simulink model "UART"  (R2025a)
settings: Solver=FixedStepAuto  StartTime=0.0  StopTime=10  FixedStep=1e-6  RelTol=1e-3
undefined symbols (not defined in the file): Bit_1, Bit_2, Bit_3, Bit_4, Bit_5, Bit_6, Bit_7, Bit_8
libraries: simulink_extras x158, fl_lib x17, nesl_utility x8, simulink x7
(part 6 of 6)

== system UART/Subsystem1/Baudrate Generator/BPS/Subsystem1 ==
  Data : Inport
  Store : Inport  Port=2
  Clock : Inport  Port=3
  Clear : Inport  Port=4
  AND : Logic  IconShape=distinctive  AllPortsSameDT=off  OutDataTypeStr=boolean
  AND1 : Logic  IconShape=distinctive  AllPortsSameDT=off  OutDataTypeStr=boolean
  D Flip-Flop : simulink_extras/Flip Flops/D Flip-Flop
  NOT : Logic  Operator=NOT  IconShape=distinctive  AllPortsSameDT=off  OutDataTypeStr=boolean
  NOT1 : Logic  Operator=NOT  IconShape=distinctive  AllPortsSameDT=off  OutDataTypeStr=boolean
  OR : Logic  Operator=OR  IconShape=distinctive  AllPortsSameDT=off  OutDataTypeStr=boolean
  Q : Outport
  !Q : Outport  Port=2
  wires:
  AND1/1 -> OR/2
  AND/1 -> OR/1
  D Flip-Flop/1 -> Q/1, AND1/2
  NOT/1 -> AND1/1
  Store/1 -> AND/2, NOT/1
  Clock/1 -> D Flip-Flop/2
  Data/1 -> AND/1
  OR/1 -> D Flip-Flop/1
  D Flip-Flop/2 -> !Q/1
  Clear/1 -> NOT1/1
  NOT1/1 -> D Flip-Flop/3

== system UART/Subsystem1/Baudrate Generator/BPS/Subsystem2 ==
  Data : Inport
  Store : Inport  Port=2
  Clock : Inport  Port=3
  Clear : Inport  Port=4
  AND : Logic  IconShape=distinctive  AllPortsSameDT=off  OutDataTypeStr=boolean
  AND1 : Logic  IconShape=distinctive  AllPortsSameDT=off  OutDataTypeStr=boolean
  D Flip-Flop : simulink_extras/Flip Flops/D Flip-Flop
  NOT : Logic  Operator=NOT  IconShape=distinctive  AllPortsSameDT=off  OutDataTypeStr=boolean
  NOT1 : Logic  Operator=NOT  IconShape=distinctive  AllPortsSameDT=off  OutDataTypeStr=boolean
  OR : Logic  Operator=OR  IconShape=distinctive  AllPortsSameDT=off  OutDataTypeStr=boolean
  Q : Outport
  !Q : Outport  Port=2
  wires:
  AND1/1 -> OR/2
  AND/1 -> OR/1
  D Flip-Flop/1 -> Q/1, AND1/2
  NOT/1 -> AND1/1
  Store/1 -> AND/2, NOT/1
  Clock/1 -> D Flip-Flop/2
  Data/1 -> AND/1
  OR/1 -> D Flip-Flop/1
  D Flip-Flop/2 -> !Q/1
  Clear/1 -> NOT1/1
  NOT1/1 -> D Flip-Flop/3

== system UART/Subsystem1/Baudrate Generator/BPS/Subsystem3 ==
  Data : Inport
  Store : Inport  Port=2
  Clock : Inport  Port=3
  Clear : Inport  Port=4
  AND : Logic  IconShape=distinctive  AllPortsSameDT=off  OutDataTypeStr=boolean
  AND1 : Logic  IconShape=distinctive  AllPortsSameDT=off  OutDataTypeStr=boolean
  D Flip-Flop : simulink_extras/Flip Flops/D Flip-Flop
  NOT : Logic  Operator=NOT  IconShape=distinctive  AllPortsSameDT=off  OutDataTypeStr=boolean
  NOT1 : Logic  Operator=NOT  IconShape=distinctive  AllPortsSameDT=off  OutDataTypeStr=boolean
  OR : Logic  Operator=OR  IconShape=distinctive  AllPortsSameDT=off  OutDataTypeStr=boolean
  Q : Outport
  !Q : Outport  Port=2
  wires:
  AND1/1 -> OR/2
  AND/1 -> OR/1
  D Flip-Flop/1 -> Q/1, AND1/2
  NOT/1 -> AND1/1
  Store/1 -> AND/2, NOT/1
  Clock/1 -> D Flip-Flop/2
  Data/1 -> AND/1
  OR/1 -> D Flip-Flop/1
  D Flip-Flop/2 -> !Q/1
  Clear/1 -> NOT1/1
  NOT1/1 -> D Flip-Flop/3

== system UART/Subsystem1/Baudrate Generator/BPS/Subsystem4 ==
  Data : Inport
  Store : Inport  Port=2
  Clock : Inport  Port=3
  Clear : Inport  Port=4
  AND : Logic  IconShape=distinctive  AllPortsSameDT=off  OutDataTypeStr=boolean
  AND1 : Logic  IconShape=distinctive  AllPortsSameDT=off  OutDataTypeStr=boolean
  D Flip-Flop : simulink_extras/Flip Flops/D Flip-Flop
  NOT : Logic  Operator=NOT  IconShape=distinctive  AllPortsSameDT=off  OutDataTypeStr=boolean
  NOT1 : Logic  Operator=NOT  IconShape=distinctive  AllPortsSameDT=off  OutDataTypeStr=boolean
  OR : Logic  Operator=OR  IconShape=distinctive  AllPortsSameDT=off  OutDataTypeStr=boolean
  Q : Outport
  !Q : Outport  Port=2
  wires:
  AND1/1 -> OR/2
  AND/1 -> OR/1
  D Flip-Flop/1 -> Q/1, AND1/2
  NOT/1 -> AND1/1
  Store/1 -> AND/2, NOT/1
  Clock/1 -> D Flip-Flop/2
  Data/1 -> AND/1
  OR/1 -> D Flip-Flop/1
  D Flip-Flop/2 -> !Q/1
  Clear/1 -> NOT1/1
  NOT1/1 -> D Flip-Flop/3

== system UART/Subsystem1/Baudrate Generator/BPS/Subsystem5 ==
  Data : Inport
  Store : Inport  Port=2
  Clock : Inport  Port=3
  Clear : Inport  Port=4
  AND : Logic  IconShape=distinctive  AllPortsSameDT=off  OutDataTypeStr=boolean
  AND1 : Logic  IconShape=distinctive  AllPortsSameDT=off  OutDataTypeStr=boolean
  D Flip-Flop : simulink_extras/Flip Flops/D Flip-Flop
  NOT : Logic  Operator=NOT  IconShape=distinctive  AllPortsSameDT=off  OutDataTypeStr=boolean
  NOT1 : Logic  Operator=NOT  IconShape=distinctive  AllPortsSameDT=off  OutDataTypeStr=boolean
  OR : Logic  Operator=OR  IconShape=distinctive  AllPortsSameDT=off  OutDataTypeStr=boolean
  Q : Outport
  !Q : Outport  Port=2
  wires:
  AND1/1 -> OR/2
  AND/1 -> OR/1
  D Flip-Flop/1 -> Q/1, AND1/2
  NOT/1 -> AND1/1
  Store/1 -> AND/2, NOT/1
  Clock/1 -> D Flip-Flop/2
  Data/1 -> AND/1
  OR/1 -> D Flip-Flop/1
  D Flip-Flop/2 -> !Q/1
  Clear/1 -> NOT1/1
  NOT1/1 -> D Flip-Flop/3

== system UART/Subsystem1/Baudrate Generator/BPS/Subsystem6 ==
  Data : Inport
  Store : Inport  Port=2
  Clock : Inport  Port=3
  Clear : Inport  Port=4
  AND : Logic  IconShape=distinctive  AllPortsSameDT=off  OutDataTypeStr=boolean
  AND1 : Logic  IconShape=distinctive  AllPortsSameDT=off  OutDataTypeStr=boolean
  D Flip-Flop : simulink_extras/Flip Flops/D Flip-Flop
  NOT : Logic  Operator=NOT  IconShape=distinctive  AllPortsSameDT=off  OutDataTypeStr=boolean
  NOT1 : Logic  Operator=NOT  IconShape=distinctive  AllPortsSameDT=off  OutDataTypeStr=boolean
  OR : Logic  Operator=OR  IconShape=distinctive  AllPortsSameDT=off  OutDataTypeStr=boolean
  Q : Outport
  !Q : Outport  Port=2
  wires:
  AND1/1 -> OR/2
  AND/1 -> OR/1
  D Flip-Flop/1 -> Q/1, AND1/2
  NOT/1 -> AND1/1
  Store/1 -> AND/2, NOT/1
  Clock/1 -> D Flip-Flop/2
  Data/1 -> AND/1
  OR/1 -> D Flip-Flop/1
  D Flip-Flop/2 -> !Q/1
  Clear/1 -> NOT1/1
  NOT1/1 -> D Flip-Flop/3

== system UART/Subsystem1/Baudrate Generator/BPS/Subsystem7 ==
  Data : Inport
  Store : Inport  Port=2
  Clock : Inport  Port=3
  Clear : Inport  Port=4
  AND : Logic  IconShape=distinctive  AllPortsSameDT=off  OutDataTypeStr=boolean
  AND1 : Logic  IconShape=distinctive  AllPortsSameDT=off  OutDataTypeStr=boolean
  D Flip-Flop : simulink_extras/Flip Flops/D Flip-Flop
  NOT : Logic  Operator=NOT  IconShape=distinctive  AllPortsSameDT=off  OutDataTypeStr=boolean
  NOT1 : Logic  Operator=NOT  IconShape=distinctive  AllPortsSameDT=off  OutDataTypeStr=boolean
  OR : Logic  Operator=OR  IconShape=distinctive  AllPortsSameDT=off  OutDataTypeStr=boolean
  Q : Outport
  !Q : Outport  Port=2
  wires:
  AND1/1 -> OR/2
  AND/1 -> OR/1
  D Flip-Flop/1 -> Q/1, AND1/2
  NOT/1 -> AND1/1
  Store/1 -> AND/2, NOT/1
  Clock/1 -> D Flip-Flop/2
  Data/1 -> AND/1
  OR/1 -> D Flip-Flop/1
  D Flip-Flop/2 -> !Q/1
  Clear/1 -> NOT1/1
  NOT1/1 -> D Flip-Flop/3

== system UART/Subsystem1/Baudrate Generator/BPS/Subsystem8 ==
  Data : Inport
  Store : Inport  Port=2
  Clock : Inport  Port=3
  Clear : Inport  Port=4
  AND : Logic  IconShape=distinctive  AllPortsSameDT=off  OutDataTypeStr=boolean
  AND1 : Logic  IconShape=distinctive  AllPortsSameDT=off  OutDataTypeStr=boolean
  D Flip-Flop : simulink_extras/Flip Flops/D Flip-Flop
  NOT : Logic  Operator=NOT  IconShape=distinctive  AllPortsSameDT=off  OutDataTypeStr=boolean
  NOT1 : Logic  Operator=NOT  IconShape=distinctive  AllPortsSameDT=off  OutDataTypeStr=boolean
  OR : Logic  Operator=OR  IconShape=distinctive  AllPortsSameDT=off  OutDataTypeStr=boolean
  Q : Outport
  !Q : Outport  Port=2
  wires:
  AND1/1 -> OR/2
  AND/1 -> OR/1
  D Flip-Flop/1 -> Q/1, AND1/2
  NOT/1 -> AND1/1
  Store/1 -> AND/2, NOT/1
  Clock/1 -> D Flip-Flop/2
  Data/1 -> AND/1
  OR/1 -> D Flip-Flop/1
  D Flip-Flop/2 -> !Q/1
  Clear/1 -> NOT1/1
  NOT1/1 -> D Flip-Flop/3

== system UART/Subsystem1/Baudrate Generator/BR/Subsystem1 ==
  Data : Inport
  Store : Inport  Port=2
  Clock : Inport  Port=3
  Clear : Inport  Port=4
  AND : Logic  IconShape=distinctive  AllPortsSameDT=off  OutDataTypeStr=boolean
  AND1 : Logic  IconShape=distinctive  AllPortsSameDT=off  OutDataTypeStr=boolean
  D Flip-Flop : simulink_extras/Flip Flops/D Flip-Flop
  NOT : Logic  Operator=NOT  IconShape=distinctive  AllPortsSameDT=off  OutDataTypeStr=boolean
  NOT1 : Logic  Operator=NOT  IconShape=distinctive  AllPortsSameDT=off  OutDataTypeStr=boolean
  OR : Logic  Operator=OR  IconShape=distinctive  AllPortsSameDT=off  OutDataTypeStr=boolean
  Q : Outport
  !Q : Outport  Port=2
  wires:
  AND1/1 -> OR/2
  AND/1 -> OR/1
  D Flip-Flop/1 -> Q/1, AND1/2
  NOT/1 -> AND1/1
  Store/1 -> AND/2, NOT/1
  Clock/1 -> D Flip-Flop/2
  Data/1 -> AND/1
  OR/1 -> D Flip-Flop/1
  D Flip-Flop/2 -> !Q/1
  Clear/1 -> NOT1/1
  NOT1/1 -> D Flip-Flop/3

== system UART/Subsystem1/Baudrate Generator/BR/Subsystem2 ==
  Data : Inport
  Store : Inport  Port=2
  Clock : Inport  Port=3
  Clear : Inport  Port=4
  AND : Logic  IconShape=distinctive  AllPortsSameDT=off  OutDataTypeStr=boolean
  AND1 : Logic  IconShape=distinctive  AllPortsSameDT=off  OutDataTypeStr=boolean
  D Flip-Flop : simulink_extras/Flip Flops/D Flip-Flop
  NOT : Logic  Operator=NOT  IconShape=distinctive  AllPortsSameDT=off  OutDataTypeStr=boolean
  NOT1 : Logic  Operator=NOT  IconShape=distinctive  AllPortsSameDT=off  OutDataTypeStr=boolean
  OR : Logic  Operator=OR  IconShape=distinctive  AllPortsSameDT=off  OutDataTypeStr=boolean
  Q : Outport
  !Q : Outport  Port=2
  wires:
  AND1/1 -> OR/2
  AND/1 -> OR/1
  D Flip-Flop/1 -> Q/1, AND1/2
  NOT/1 -> AND1/1
  Store/1 -> AND/2, NOT/1
  Clock/1 -> D Flip-Flop/2
  Data/1 -> AND/1
  OR/1 -> D Flip-Flop/1
  D Flip-Flop/2 -> !Q/1
  Clear/1 -> NOT1/1
  NOT1/1 -> D Flip-Flop/3

== system UART/Subsystem1/Baudrate Generator/BR/Subsystem3 ==
  Data : Inport
  Store : Inport  Port=2
  Clock : Inport  Port=3
  Clear : Inport  Port=4
  AND : Logic  IconShape=distinctive  AllPortsSameDT=off  OutDataTypeStr=boolean
  AND1 : Logic  IconShape=distinctive  AllPortsSameDT=off  OutDataTypeStr=boolean
  D Flip-Flop : simulink_extras/Flip Flops/D Flip-Flop
  NOT : Logic  Operator=NOT  IconShape=distinctive  AllPortsSameDT=off  OutDataTypeStr=boolean
  NOT1 : Logic  Operator=NOT  IconShape=distinctive  AllPortsSameDT=off  OutDataTypeStr=boolean
  OR : Logic  Operator=OR  IconShape=distinctive  AllPortsSameDT=off  OutDataTypeStr=boolean
  Q : Outport
  !Q : Outport  Port=2
  wires:
  AND1/1 -> OR/2
  AND/1 -> OR/1
  D Flip-Flop/1 -> Q/1, AND1/2
  NOT/1 -> AND1/1
  Store/1 -> AND/2, NOT/1
  Clock/1 -> D Flip-Flop/2
  Data/1 -> AND/1
  OR/1 -> D Flip-Flop/1
  D Flip-Flop/2 -> !Q/1
  Clear/1 -> NOT1/1
  NOT1/1 -> D Flip-Flop/3

== system UART/Subsystem1/Baudrate Generator/BR/Subsystem4 ==
  Data : Inport
  Store : Inport  Port=2
  Clock : Inport  Port=3
  Clear : Inport  Port=4
  AND : Logic  IconShape=distinctive  AllPortsSameDT=off  OutDataTypeStr=boolean
  AND1 : Logic  IconShape=distinctive  AllPortsSameDT=off  OutDataTypeStr=boolean
  D Flip-Flop : simulink_extras/Flip Flops/D Flip-Flop
  NOT : Logic  Operator=NOT  IconShape=distinctive  AllPortsSameDT=off  OutDataTypeStr=boolean
  NOT1 : Logic  Operator=NOT  IconShape=distinctive  AllPortsSameDT=off  OutDataTypeStr=boolean
  OR : Logic  Operator=OR  IconShape=distinctive  AllPortsSameDT=off  OutDataTypeStr=boolean
  Q : Outport
  !Q : Outport  Port=2
  wires:
  AND1/1 -> OR/2
  AND/1 -> OR/1
  D Flip-Flop/1 -> Q/1, AND1/2
  NOT/1 -> AND1/1
  Store/1 -> AND/2, NOT/1
  Clock/1 -> D Flip-Flop/2
  Data/1 -> AND/1
  OR/1 -> D Flip-Flop/1
  D Flip-Flop/2 -> !Q/1
  Clear/1 -> NOT1/1
  NOT1/1 -> D Flip-Flop/3

== system UART/Subsystem1/Baudrate Generator/BR/Subsystem5 ==
  Data : Inport
  Store : Inport  Port=2
  Clock : Inport  Port=3
  Clear : Inport  Port=4
  AND : Logic  IconShape=distinctive  AllPortsSameDT=off  OutDataTypeStr=boolean
  AND1 : Logic  IconShape=distinctive  AllPortsSameDT=off  OutDataTypeStr=boolean
  D Flip-Flop : simulink_extras/Flip Flops/D Flip-Flop
  NOT : Logic  Operator=NOT  IconShape=distinctive  AllPortsSameDT=off  OutDataTypeStr=boolean
  NOT1 : Logic  Operator=NOT  IconShape=distinctive  AllPortsSameDT=off  OutDataTypeStr=boolean
  OR : Logic  Operator=OR  IconShape=distinctive  AllPortsSameDT=off  OutDataTypeStr=boolean
  Q : Outport
  !Q : Outport  Port=2
  wires:
  AND1/1 -> OR/2
  AND/1 -> OR/1
  D Flip-Flop/1 -> Q/1, AND1/2
  NOT/1 -> AND1/1
  Store/1 -> AND/2, NOT/1
  Clock/1 -> D Flip-Flop/2
  Data/1 -> AND/1
  OR/1 -> D Flip-Flop/1
  D Flip-Flop/2 -> !Q/1
  Clear/1 -> NOT1/1
  NOT1/1 -> D Flip-Flop/3

== system UART/Subsystem1/Baudrate Generator/BR/Subsystem6 ==
  Data : Inport
  Store : Inport  Port=2
  Clock : Inport  Port=3
  Clear : Inport  Port=4
  AND : Logic  IconShape=distinctive  AllPortsSameDT=off  OutDataTypeStr=boolean
  AND1 : Logic  IconShape=distinctive  AllPortsSameDT=off  OutDataTypeStr=boolean
  D Flip-Flop : simulink_extras/Flip Flops/D Flip-Flop
  NOT : Logic  Operator=NOT  IconShape=distinctive  AllPortsSameDT=off  OutDataTypeStr=boolean
  NOT1 : Logic  Operator=NOT  IconShape=distinctive  AllPortsSameDT=off  OutDataTypeStr=boolean
  OR : Logic  Operator=OR  IconShape=distinctive  AllPortsSameDT=off  OutDataTypeStr=boolean
  Q : Outport
  !Q : Outport  Port=2
  wires:
  AND1/1 -> OR/2
  AND/1 -> OR/1
  D Flip-Flop/1 -> Q/1, AND1/2
  NOT/1 -> AND1/1
  Store/1 -> AND/2, NOT/1
  Clock/1 -> D Flip-Flop/2
  Data/1 -> AND/1
  OR/1 -> D Flip-Flop/1
  D Flip-Flop/2 -> !Q/1
  Clear/1 -> NOT1/1
  NOT1/1 -> D Flip-Flop/3

== system UART/Subsystem1/Baudrate Generator/BR/Subsystem7 ==
  Data : Inport
  Store : Inport  Port=2
  Clock : Inport  Port=3
  Clear : Inport  Port=4
  AND : Logic  IconShape=distinctive  AllPortsSameDT=off  OutDataTypeStr=boolean
  AND1 : Logic  IconShape=distinctive  AllPortsSameDT=off  OutDataTypeStr=boolean
  D Flip-Flop : simulink_extras/Flip Flops/D Flip-Flop
  NOT : Logic  Operator=NOT  IconShape=distinctive  AllPortsSameDT=off  OutDataTypeStr=boolean
  NOT1 : Logic  Operator=NOT  IconShape=distinctive  AllPortsSameDT=off  OutDataTypeStr=boolean
  OR : Logic  Operator=OR  IconShape=distinctive  AllPortsSameDT=off  OutDataTypeStr=boolean
  Q : Outport
  !Q : Outport  Port=2
  wires:
  AND1/1 -> OR/2
  AND/1 -> OR/1
  D Flip-Flop/1 -> Q/1, AND1/2
  NOT/1 -> AND1/1
  Store/1 -> AND/2, NOT/1
  Clock/1 -> D Flip-Flop/2
  Data/1 -> AND/1
  OR/1 -> D Flip-Flop/1
  D Flip-Flop/2 -> !Q/1
  Clear/1 -> NOT1/1
  NOT1/1 -> D Flip-Flop/3

== system UART/Subsystem1/Baudrate Generator/BR/Subsystem8 ==
  Data : Inport
  Store : Inport  Port=2
  Clock : Inport  Port=3
  Clear : Inport  Port=4
  AND : Logic  IconShape=distinctive  AllPortsSameDT=off  OutDataTypeStr=boolean
  AND1 : Logic  IconShape=distinctive  AllPortsSameDT=off  OutDataTypeStr=boolean
  D Flip-Flop : simulink_extras/Flip Flops/D Flip-Flop
  NOT : Logic  Operator=NOT  IconShape=distinctive  AllPortsSameDT=off  OutDataTypeStr=boolean
  NOT1 : Logic  Operator=NOT  IconShape=distinctive  AllPortsSameDT=off  OutDataTypeStr=boolean
  OR : Logic  Operator=OR  IconShape=distinctive  AllPortsSameDT=off  OutDataTypeStr=boolean
  Q : Outport
  !Q : Outport  Port=2
  wires:
  AND1/1 -> OR/2
  AND/1 -> OR/1
  D Flip-Flop/1 -> Q/1, AND1/2
  NOT/1 -> AND1/1
  Store/1 -> AND/2, NOT/1
  Clock/1 -> D Flip-Flop/2
  Data/1 -> AND/1
  OR/1 -> D Flip-Flop/1
  D Flip-Flop/2 -> !Q/1
  Clear/1 -> NOT1/1
  NOT1/1 -> D Flip-Flop/3

== system UART/Subsystem1/Baudrate Generator/Counter/Half Adder ==
  A : Inport
  "B " : Inport  Port=2
  AND : Logic  IconShape=distinctive  AllPortsSameDT=off  OutDataTypeStr=boolean
  XOR : Logic  Operator=XOR  IconShape=distinctive  AllPortsSameDT=off  OutDataTypeStr=boolean
  Sum : Outport
  Carry : Outport  Port=2
  wires:
  A/1 -> AND/1, XOR/1
  "B "/1 -> XOR/2, AND/2
  XOR/1 -> Sum/1
  AND/1 -> Carry/1

== system UART/Subsystem1/Baudrate Generator/Counter/Half Adder1 ==
  A : Inport
  "B " : Inport  Port=2
  AND : Logic  IconShape=distinctive  AllPortsSameDT=off  OutDataTypeStr=boolean
  XOR : Logic  Operator=XOR  IconShape=distinctive  AllPortsSameDT=off  OutDataTypeStr=boolean
  Sum : Outport
  Carry : Outport  Port=2
  wires:
  A/1 -> AND/1, XOR/1
  "B "/1 -> XOR/2, AND/2
  XOR/1 -> Sum/1
  AND/1 -> Carry/1

== system UART/Subsystem1/Baudrate Generator/Counter/Half Adder2 ==
  A : Inport
  "B " : Inport  Port=2
  AND : Logic  IconShape=distinctive  AllPortsSameDT=off  OutDataTypeStr=boolean
  XOR : Logic  Operator=XOR  IconShape=distinctive  AllPortsSameDT=off  OutDataTypeStr=boolean
  Sum : Outport
  Carry : Outport  Port=2
  wires:
  A/1 -> AND/1, XOR/1
  "B "/1 -> XOR/2, AND/2
  XOR/1 -> Sum/1
  AND/1 -> Carry/1

== system UART/Subsystem1/Baudrate Generator/Counter/Half Adder3 ==
  A : Inport
  "B " : Inport  Port=2
  AND : Logic  IconShape=distinctive  AllPortsSameDT=off  OutDataTypeStr=boolean
  XOR : Logic  Operator=XOR  IconShape=distinctive  AllPortsSameDT=off  OutDataTypeStr=boolean
  Sum : Outport
  Carry : Outport  Port=2
  wires:
  A/1 -> AND/1, XOR/1
  "B "/1 -> XOR/2, AND/2
  XOR/1 -> Sum/1
  AND/1 -> Carry/1

== system UART/Subsystem1/Baudrate Generator/Counter/Half Adder4 ==
  A : Inport
  "B " : Inport  Port=2
  AND : Logic  IconShape=distinctive  AllPortsSameDT=off  OutDataTypeStr=boolean
  XOR : Logic  Operator=XOR  IconShape=distinctive  AllPortsSameDT=off  OutDataTypeStr=boolean
  Sum : Outport
  Carry : Outport  Port=2
  wires:
  A/1 -> AND/1, XOR/1
  "B "/1 -> XOR/2, AND/2
  XOR/1 -> Sum/1
  AND/1 -> Carry/1

== system UART/Subsystem1/Baudrate Generator/Counter/Half Adder5 ==
  A : Inport
  "B " : Inport  Port=2
  AND : Logic  IconShape=distinctive  AllPortsSameDT=off  OutDataTypeStr=boolean
  XOR : Logic  Operator=XOR  IconShape=distinctive  AllPortsSameDT=off  OutDataTypeStr=boolean
  Sum : Outport
  Carry : Outport  Port=2
  wires:
  A/1 -> AND/1, XOR/1
  "B "/1 -> XOR/2, AND/2
  XOR/1 -> Sum/1
  AND/1 -> Carry/1

== system UART/Subsystem1/Baudrate Generator/Counter/Half Adder6 ==
  A : Inport
  "B " : Inport  Port=2
  XOR : Logic  Operator=XOR  IconShape=distinctive  AllPortsSameDT=off  OutDataTypeStr=boolean
  Sum : Outport
  wires:
  A/1 -> XOR/1
  "B "/1 -> XOR/2
  XOR/1 -> Sum/1

== system UART/Subsystem1/Baudrate Generator/Counter/Half Adder7 ==
  A : Inport
  "B " : Inport  Port=2
  AND : Logic  IconShape=distinctive  AllPortsSameDT=off  OutDataTypeStr=boolean
  XOR : Logic  Operator=XOR  IconShape=distinctive  AllPortsSameDT=off  OutDataTypeStr=boolean
  Sum : Outport
  Carry : Outport  Port=2
  wires:
  A/1 -> AND/1, XOR/1
  "B "/1 -> XOR/2, AND/2
  XOR/1 -> Sum/1
  AND/1 -> Carry/1

== system UART/Subsystem1/Baudrate Generator/Counter1/Half Adder ==
  A : Inport
  "B " : Inport  Port=2
  AND : Logic  IconShape=distinctive  AllPortsSameDT=off  OutDataTypeStr=boolean
  XOR : Logic  Operator=XOR  IconShape=distinctive  AllPortsSameDT=off  OutDataTypeStr=boolean
  Sum : Outport
  Carry : Outport  Port=2
  wires:
  A/1 -> AND/1, XOR/1
  "B "/1 -> XOR/2, AND/2
  XOR/1 -> Sum/1
  AND/1 -> Carry/1

== system UART/Subsystem1/Baudrate Generator/Counter1/Half Adder1 ==
  A : Inport
  "B " : Inport  Port=2
  AND : Logic  IconShape=distinctive  AllPortsSameDT=off  OutDataTypeStr=boolean
  XOR : Logic  Operator=XOR  IconShape=distinctive  AllPortsSameDT=off  OutDataTypeStr=boolean
  Sum : Outport
  Carry : Outport  Port=2
  wires:
  A/1 -> AND/1, XOR/1
  "B "/1 -> XOR/2, AND/2
  XOR/1 -> Sum/1
  AND/1 -> Carry/1

== system UART/Subsystem1/Baudrate Generator/Counter1/Half Adder2 ==
  A : Inport
  "B " : Inport  Port=2
  AND : Logic  IconShape=distinctive  AllPortsSameDT=off  OutDataTypeStr=boolean
  XOR : Logic  Operator=XOR  IconShape=distinctive  AllPortsSameDT=off  OutDataTypeStr=boolean
  Sum : Outport
  Carry : Outport  Port=2
  wires:
  A/1 -> AND/1, XOR/1
  "B "/1 -> XOR/2, AND/2
  XOR/1 -> Sum/1
  AND/1 -> Carry/1

== system UART/Subsystem1/Baudrate Generator/Counter1/Half Adder3 ==
  A : Inport
  "B " : Inport  Port=2
  AND : Logic  IconShape=distinctive  AllPortsSameDT=off  OutDataTypeStr=boolean
  XOR : Logic  Operator=XOR  IconShape=distinctive  AllPortsSameDT=off  OutDataTypeStr=boolean
  Sum : Outport
  Carry : Outport  Port=2
  wires:
  A/1 -> AND/1, XOR/1
  "B "/1 -> XOR/2, AND/2
  XOR/1 -> Sum/1
  AND/1 -> Carry/1

== system UART/Subsystem1/Baudrate Generator/Counter1/Half Adder4 ==
  A : Inport
  "B " : Inport  Port=2
  AND : Logic  IconShape=distinctive  AllPortsSameDT=off  OutDataTypeStr=boolean
  XOR : Logic  Operator=XOR  IconShape=distinctive  AllPortsSameDT=off  OutDataTypeStr=boolean
  Sum : Outport
  Carry : Outport  Port=2
  wires:
  A/1 -> AND/1, XOR/1
  "B "/1 -> XOR/2, AND/2
  XOR/1 -> Sum/1
  AND/1 -> Carry/1

== system UART/Subsystem1/Baudrate Generator/Counter1/Half Adder5 ==
  A : Inport
  "B " : Inport  Port=2
  AND : Logic  IconShape=distinctive  AllPortsSameDT=off  OutDataTypeStr=boolean
  XOR : Logic  Operator=XOR  IconShape=distinctive  AllPortsSameDT=off  OutDataTypeStr=boolean
  Sum : Outport
  Carry : Outport  Port=2
  wires:
  A/1 -> AND/1, XOR/1
  "B "/1 -> XOR/2, AND/2
  XOR/1 -> Sum/1
  AND/1 -> Carry/1

== system UART/Subsystem1/Baudrate Generator/Counter1/Half Adder6 ==
  A : Inport
  "B " : Inport  Port=2
  XOR : Logic  Operator=XOR  IconShape=distinctive  AllPortsSameDT=off  OutDataTypeStr=boolean
  Sum : Outport
  wires:
  A/1 -> XOR/1
  "B "/1 -> XOR/2
  XOR/1 -> Sum/1

== system UART/Subsystem1/Baudrate Generator/Counter1/Half Adder7 ==
  A : Inport
  "B " : Inport  Port=2
  AND : Logic  IconShape=distinctive  AllPortsSameDT=off  OutDataTypeStr=boolean
  XOR : Logic  Operator=XOR  IconShape=distinctive  AllPortsSameDT=off  OutDataTypeStr=boolean
  Sum : Outport
  Carry : Outport  Port=2
  wires:
  A/1 -> AND/1, XOR/1
  "B "/1 -> XOR/2, AND/2
  XOR/1 -> Sum/1
  AND/1 -> Carry/1

== system UART/Rx Only/Baudrate Generator/BaudTimer/Counter/Half Adder ==
  A : Inport
  "B " : Inport  Port=2
  AND : Logic  IconShape=distinctive  AllPortsSameDT=off  OutDataTypeStr=boolean
  XOR : Logic  Operator=XOR  IconShape=distinctive  AllPortsSameDT=off  OutDataTypeStr=boolean
  Sum : Outport
  Carry : Outport  Port=2
  wires:
  A/1 -> AND/1, XOR/1
  "B "/1 -> XOR/2, AND/2
  XOR/1 -> Sum/1
  AND/1 -> Carry/1

== system UART/Rx Only/Baudrate Generator/BaudTimer/Counter/Half Adder1 ==
  A : Inport
  "B " : Inport  Port=2
  AND : Logic  IconShape=distinctive  AllPortsSameDT=off  OutDataTypeStr=boolean
  XOR : Logic  Operator=XOR  IconShape=distinctive  AllPortsSameDT=off  OutDataTypeStr=boolean
  Sum : Outport
  Carry : Outport  Port=2
  wires:
  A/1 -> AND/1, XOR/1
  "B "/1 -> XOR/2, AND/2
  XOR/1 -> Sum/1
  AND/1 -> Carry/1

== system UART/Rx Only/Baudrate Generator/BaudTimer/Counter/Half Adder2 ==
  A : Inport
  "B " : Inport  Port=2
  AND : Logic  IconShape=distinctive  AllPortsSameDT=off  OutDataTypeStr=boolean
  XOR : Logic  Operator=XOR  IconShape=distinctive  AllPortsSameDT=off  OutDataTypeStr=boolean
  Sum : Outport
  Carry : Outport  Port=2
  wires:
  A/1 -> AND/1, XOR/1
  "B "/1 -> XOR/2, AND/2
  XOR/1 -> Sum/1
  AND/1 -> Carry/1

== system UART/Rx Only/Baudrate Generator/BaudTimer/Counter/Half Adder3 ==
  A : Inport
  "B " : Inport  Port=2
  AND : Logic  IconShape=distinctive  AllPortsSameDT=off  OutDataTypeStr=boolean
  XOR : Logic  Operator=XOR  IconShape=distinctive  AllPortsSameDT=off  OutDataTypeStr=boolean
  Sum : Outport
  Carry : Outport  Port=2
  wires:
  A/1 -> AND/1, XOR/1
  "B "/1 -> XOR/2, AND/2
  XOR/1 -> Sum/1
  AND/1 -> Carry/1

== system UART/Rx Only/Baudrate Generator/BaudTimer/Counter/Half Adder4 ==
  A : Inport
  "B " : Inport  Port=2
  AND : Logic  IconShape=distinctive  AllPortsSameDT=off  OutDataTypeStr=boolean
  XOR : Logic  Operator=XOR  IconShape=distinctive  AllPortsSameDT=off  OutDataTypeStr=boolean
  Sum : Outport
  Carry : Outport  Port=2
  wires:
  A/1 -> AND/1, XOR/1
  "B "/1 -> XOR/2, AND/2
  XOR/1 -> Sum/1
  AND/1 -> Carry/1

== system UART/Rx Only/Baudrate Generator/BaudTimer/Counter/Half Adder5 ==
  A : Inport
  "B " : Inport  Port=2
  AND : Logic  IconShape=distinctive  AllPortsSameDT=off  OutDataTypeStr=boolean
  XOR : Logic  Operator=XOR  IconShape=distinctive  AllPortsSameDT=off  OutDataTypeStr=boolean
  Sum : Outport
  Carry : Outport  Port=2
  wires:
  A/1 -> AND/1, XOR/1
  "B "/1 -> XOR/2, AND/2
  XOR/1 -> Sum/1
  AND/1 -> Carry/1

== system UART/Rx Only/Baudrate Generator/BaudTimer/Counter/Half Adder6 ==
  A : Inport
  "B " : Inport  Port=2
  XOR : Logic  Operator=XOR  IconShape=distinctive  AllPortsSameDT=off  OutDataTypeStr=boolean
  Sum : Outport
  wires:
  A/1 -> XOR/1
  "B "/1 -> XOR/2
  XOR/1 -> Sum/1

== system UART/Rx Only/Baudrate Generator/BaudTimer/Counter/Half Adder7 ==
  A : Inport
  "B " : Inport  Port=2
  AND : Logic  IconShape=distinctive  AllPortsSameDT=off  OutDataTypeStr=boolean
  XOR : Logic  Operator=XOR  IconShape=distinctive  AllPortsSameDT=off  OutDataTypeStr=boolean
  Sum : Outport
  Carry : Outport  Port=2
  wires:
  A/1 -> AND/1, XOR/1
  "B "/1 -> XOR/2, AND/2
  XOR/1 -> Sum/1
  AND/1 -> Carry/1

== system UART/Rx Only/Baudrate Generator/BaudTimer/Counter1/Half Adder ==
  A : Inport
  "B " : Inport  Port=2
  AND : Logic  IconShape=distinctive  AllPortsSameDT=off  OutDataTypeStr=boolean
  XOR : Logic  Operator=XOR  IconShape=distinctive  AllPortsSameDT=off  OutDataTypeStr=boolean
  Sum : Outport
  Carry : Outport  Port=2
  wires:
  A/1 -> AND/1, XOR/1
  "B "/1 -> XOR/2, AND/2
  XOR/1 -> Sum/1
  AND/1 -> Carry/1

== system UART/Rx Only/Baudrate Generator/BaudTimer/Counter1/Half Adder1 ==
  A : Inport
  "B " : Inport  Port=2
  AND : Logic  IconShape=distinctive  AllPortsSameDT=off  OutDataTypeStr=boolean
  XOR : Logic  Operator=XOR  IconShape=distinctive  AllPortsSameDT=off  OutDataTypeStr=boolean
  Sum : Outport
  Carry : Outport  Port=2
  wires:
  A/1 -> AND/1, XOR/1
  "B "/1 -> XOR/2, AND/2
  XOR/1 -> Sum/1
  AND/1 -> Carry/1

== system UART/Rx Only/Baudrate Generator/BaudTimer/Counter1/Half Adder2 ==
  A : Inport
  "B " : Inport  Port=2
  AND : Logic  IconShape=distinctive  AllPortsSameDT=off  OutDataTypeStr=boolean
  XOR : Logic  Operator=XOR  IconShape=distinctive  AllPortsSameDT=off  OutDataTypeStr=boolean
  Sum : Outport
  Carry : Outport  Port=2
  wires:
  A/1 -> AND/1, XOR/1
  "B "/1 -> XOR/2, AND/2
  XOR/1 -> Sum/1
  AND/1 -> Carry/1

== system UART/Rx Only/Baudrate Generator/BaudTimer/Counter1/Half Adder3 ==
  A : Inport
  "B " : Inport  Port=2
  AND : Logic  IconShape=distinctive  AllPortsSameDT=off  OutDataTypeStr=boolean
  XOR : Logic  Operator=XOR  IconShape=distinctive  AllPortsSameDT=off  OutDataTypeStr=boolean
  Sum : Outport
  Carry : Outport  Port=2
  wires:
  A/1 -> AND/1, XOR/1
  "B "/1 -> XOR/2, AND/2
  XOR/1 -> Sum/1
  AND/1 -> Carry/1

== system UART/Rx Only/Baudrate Generator/BaudTimer/Counter1/Half Adder4 ==
  A : Inport
  "B " : Inport  Port=2
  AND : Logic  IconShape=distinctive  AllPortsSameDT=off  OutDataTypeStr=boolean
  XOR : Logic  Operator=XOR  IconShape=distinctive  AllPortsSameDT=off  OutDataTypeStr=boolean
  Sum : Outport
  Carry : Outport  Port=2
  wires:
  A/1 -> AND/1, XOR/1
  "B "/1 -> XOR/2, AND/2
  XOR/1 -> Sum/1
  AND/1 -> Carry/1

== system UART/Rx Only/Baudrate Generator/BaudTimer/Counter1/Half Adder5 ==
  A : Inport
  "B " : Inport  Port=2
  AND : Logic  IconShape=distinctive  AllPortsSameDT=off  OutDataTypeStr=boolean
  XOR : Logic  Operator=XOR  IconShape=distinctive  AllPortsSameDT=off  OutDataTypeStr=boolean
  Sum : Outport
  Carry : Outport  Port=2
  wires:
  A/1 -> AND/1, XOR/1
  "B "/1 -> XOR/2, AND/2
  XOR/1 -> Sum/1
  AND/1 -> Carry/1

== system UART/Rx Only/Baudrate Generator/BaudTimer/Counter1/Half Adder6 ==
  A : Inport
  "B " : Inport  Port=2
  XOR : Logic  Operator=XOR  IconShape=distinctive  AllPortsSameDT=off  OutDataTypeStr=boolean
  Sum : Outport
  wires:
  A/1 -> XOR/1
  "B "/1 -> XOR/2
  XOR/1 -> Sum/1

== system UART/Rx Only/Baudrate Generator/BaudTimer/Counter1/Half Adder7 ==
  A : Inport
  "B " : Inport  Port=2
  AND : Logic  IconShape=distinctive  AllPortsSameDT=off  OutDataTypeStr=boolean
  XOR : Logic  Operator=XOR  IconShape=distinctive  AllPortsSameDT=off  OutDataTypeStr=boolean
  Sum : Outport
  Carry : Outport  Port=2
  wires:
  A/1 -> AND/1, XOR/1
  "B "/1 -> XOR/2, AND/2
  XOR/1 -> Sum/1
  AND/1 -> Carry/1

== system UART/Rx Only/Baudrate Generator/BaudTimer/TController/Prescaler_Controller1 ==
  StoreTReg : Inport
  TC : Inport  Port=2
  TReg : Inport  Port=3
  Enable : Inport  Port=4
  CLK : Inport  Port=5
  "CLR " : Inport  Port=6
  AND{,1..3} (4 alike) : Logic  IconShape=distinctive  AllPortsSameDT=off  OutDataTypeStr=boolean
  Delay One Step : Delay  DelayLength=1
  Demux : Demux  Outputs=8
  NOR : Logic  Operator=NOR  Inputs=8  IconShape=distinctive  AllPortsSameDT=off  OutDataTypeStr=boolean
  NOT : Logic  Operator=NOT  IconShape=distinctive  AllPortsSameDT=off  OutDataTypeStr=boolean
  NOT1 : Logic  Operator=NOT  IconShape=distinctive  AllPortsSameDT=off  OutDataTypeStr=boolean
  OR : Logic  Operator=OR  Inputs=3  IconShape=distinctive  AllPortsSameDT=off  OutDataTypeStr=boolean
  S-R Flip-Flop : simulink_extras/Flip Flops/S-R Flip-Flop  initial_condition=0
  Scope : Scope
      settings: ActiveDisplayYMinimum=-1  ActiveDisplayYMaximum=1  DataLoggingVariableName=ScopeData2
  XOR : Logic  Operator=XOR  IconShape=distinctive  AllPortsSameDT=off  OutDataTypeStr=boolean
  CLK_Next : Outport
  INC : Outport  Port=2
  TC_RST : Outport  Port=3
  wires:
  TReg/1 -> XOR/1
  Demux/1 -> NOR/1
  TC/1 -> XOR/2
  XOR/1 -> Demux/1
  Demux/2 -> NOR/2
  Demux/3 -> NOR/3
  Demux/4 -> NOR/4
  Demux/5 -> NOR/5
  Demux/6 -> NOR/6
  Demux/7 -> NOR/7
  Demux/8 -> NOR/8
  "CLR "/1 -> OR/3
  NOR/1 -> NOT/1, AND1/1
  Enable/1 -> AND1/2, AND/1
  OR/1 -> Delay One Step/1
  StoreTReg/1 -> OR/1
  AND/1 -> INC/1
  Delay One Step/1 -> AND3/1, TC_RST/1
  AND1/1 -> S-R Flip-Flop/1
  S-R Flip-Flop/1 -> AND2/2
  NOT/1 -> AND2/1
  AND2/1 -> OR/2, Scope/1, CLK_Next/1
  CLK/1 -> NOT1/1, AND/2
  AND3/1 -> S-R Flip-Flop/2
  NOT1/1 -> AND3/2

== system UART/Rx Only/Baudrate Generator/BaudTimer1/Counter/Half Adder ==
  A : Inport
  "B " : Inport  Port=2
  AND : Logic  IconShape=distinctive  AllPortsSameDT=off  OutDataTypeStr=boolean
  XOR : Logic  Operator=XOR  IconShape=distinctive  AllPortsSameDT=off  OutDataTypeStr=boolean
  Sum : Outport
  Carry : Outport  Port=2
  wires:
  A/1 -> AND/1, XOR/1
  "B "/1 -> XOR/2, AND/2
  XOR/1 -> Sum/1
  AND/1 -> Carry/1

== system UART/Rx Only/Baudrate Generator/BaudTimer1/Counter/Half Adder1 ==
  A : Inport
  "B " : Inport  Port=2
  AND : Logic  IconShape=distinctive  AllPortsSameDT=off  OutDataTypeStr=boolean
  XOR : Logic  Operator=XOR  IconShape=distinctive  AllPortsSameDT=off  OutDataTypeStr=boolean
  Sum : Outport
  Carry : Outport  Port=2
  wires:
  A/1 -> AND/1, XOR/1
  "B "/1 -> XOR/2, AND/2
  XOR/1 -> Sum/1
  AND/1 -> Carry/1

== system UART/Rx Only/Baudrate Generator/BaudTimer1/Counter/Half Adder2 ==
  A : Inport
  "B " : Inport  Port=2
  AND : Logic  IconShape=distinctive  AllPortsSameDT=off  OutDataTypeStr=boolean
  XOR : Logic  Operator=XOR  IconShape=distinctive  AllPortsSameDT=off  OutDataTypeStr=boolean
  Sum : Outport
  Carry : Outport  Port=2
  wires:
  A/1 -> AND/1, XOR/1
  "B "/1 -> XOR/2, AND/2
  XOR/1 -> Sum/1
  AND/1 -> Carry/1

== system UART/Rx Only/Baudrate Generator/BaudTimer1/Counter/Half Adder3 ==
  A : Inport
  "B " : Inport  Port=2
  AND : Logic  IconShape=distinctive  AllPortsSameDT=off  OutDataTypeStr=boolean
  XOR : Logic  Operator=XOR  IconShape=distinctive  AllPortsSameDT=off  OutDataTypeStr=boolean
  Sum : Outport
  Carry : Outport  Port=2
  wires:
  A/1 -> AND/1, XOR/1
  "B "/1 -> XOR/2, AND/2
  XOR/1 -> Sum/1
  AND/1 -> Carry/1

== system UART/Rx Only/Baudrate Generator/BaudTimer1/Counter/Half Adder4 ==
  A : Inport
  "B " : Inport  Port=2
  AND : Logic  IconShape=distinctive  AllPortsSameDT=off  OutDataTypeStr=boolean
  XOR : Logic  Operator=XOR  IconShape=distinctive  AllPortsSameDT=off  OutDataTypeStr=boolean
  Sum : Outport
  Carry : Outport  Port=2
  wires:
  A/1 -> AND/1, XOR/1
  "B "/1 -> XOR/2, AND/2
  XOR/1 -> Sum/1
  AND/1 -> Carry/1

== system UART/Rx Only/Baudrate Generator/BaudTimer1/Counter/Half Adder5 ==
  A : Inport
  "B " : Inport  Port=2
  AND : Logic  IconShape=distinctive  AllPortsSameDT=off  OutDataTypeStr=boolean
  XOR : Logic  Operator=XOR  IconShape=distinctive  AllPortsSameDT=off  OutDataTypeStr=boolean
  Sum : Outport
  Carry : Outport  Port=2
  wires:
  A/1 -> AND/1, XOR/1
  "B "/1 -> XOR/2, AND/2
  XOR/1 -> Sum/1
  AND/1 -> Carry/1

== system UART/Rx Only/Baudrate Generator/BaudTimer1/Counter/Half Adder6 ==
  A : Inport
  "B " : Inport  Port=2
  XOR : Logic  Operator=XOR  IconShape=distinctive  AllPortsSameDT=off  OutDataTypeStr=boolean
  Sum : Outport
  wires:
  A/1 -> XOR/1
  "B "/1 -> XOR/2
  XOR/1 -> Sum/1

== system UART/Rx Only/Baudrate Generator/BaudTimer1/Counter/Half Adder7 ==
  A : Inport
  "B " : Inport  Port=2
  AND : Logic  IconShape=distinctive  AllPortsSameDT=off  OutDataTypeStr=boolean
  XOR : Logic  Operator=XOR  IconShape=distinctive  AllPortsSameDT=off  OutDataTypeStr=boolean
  Sum : Outport
  Carry : Outport  Port=2
  wires:
  A/1 -> AND/1, XOR/1
  "B "/1 -> XOR/2, AND/2
  XOR/1 -> Sum/1
  AND/1 -> Carry/1

== system UART/Rx Only/Baudrate Generator/BaudTimer1/Counter1/Half Adder ==
  A : Inport
  "B " : Inport  Port=2
  AND : Logic  IconShape=distinctive  AllPortsSameDT=off  OutDataTypeStr=boolean
  XOR : Logic  Operator=XOR  IconShape=distinctive  AllPortsSameDT=off  OutDataTypeStr=boolean
  Sum : Outport
  Carry : Outport  Port=2
  wires:
  A/1 -> AND/1, XOR/1
  "B "/1 -> XOR/2, AND/2
  XOR/1 -> Sum/1
  AND/1 -> Carry/1

== system UART/Rx Only/Baudrate Generator/BaudTimer1/Counter1/Half Adder1 ==
  A : Inport
  "B " : Inport  Port=2
  AND : Logic  IconShape=distinctive  AllPortsSameDT=off  OutDataTypeStr=boolean
  XOR : Logic  Operator=XOR  IconShape=distinctive  AllPortsSameDT=off  OutDataTypeStr=boolean
  Sum : Outport
  Carry : Outport  Port=2
  wires:
  A/1 -> AND/1, XOR/1
  "B "/1 -> XOR/2, AND/2
  XOR/1 -> Sum/1
  AND/1 -> Carry/1

== system UART/Rx Only/Baudrate Generator/BaudTimer1/Counter1/Half Adder2 ==
  A : Inport
  "B " : Inport  Port=2
  AND : Logic  IconShape=distinctive  AllPortsSameDT=off  OutDataTypeStr=boolean
  XOR : Logic  Operator=XOR  IconShape=distinctive  AllPortsSameDT=off  OutDataTypeStr=boolean
  Sum : Outport
  Carry : Outport  Port=2
  wires:
  A/1 -> AND/1, XOR/1
  "B "/1 -> XOR/2, AND/2
  XOR/1 -> Sum/1
  AND/1 -> Carry/1

== system UART/Rx Only/Baudrate Generator/BaudTimer1/Counter1/Half Adder3 ==
  A : Inport
  "B " : Inport  Port=2
  AND : Logic  IconShape=distinctive  AllPortsSameDT=off  OutDataTypeStr=boolean
  XOR : Logic  Operator=XOR  IconShape=distinctive  AllPortsSameDT=off  OutDataTypeStr=boolean
  Sum : Outport
  Carry : Outport  Port=2
  wires:
  A/1 -> AND/1, XOR/1
  "B "/1 -> XOR/2, AND/2
  XOR/1 -> Sum/1
  AND/1 -> Carry/1

== system UART/Rx Only/Baudrate Generator/BaudTimer1/Counter1/Half Adder4 ==
  A : Inport
  "B " : Inport  Port=2
  AND : Logic  IconShape=distinctive  AllPortsSameDT=off  OutDataTypeStr=boolean
  XOR : Logic  Operator=XOR  IconShape=distinctive  AllPortsSameDT=off  OutDataTypeStr=boolean
  Sum : Outport
  Carry : Outport  Port=2
  wires:
  A/1 -> AND/1, XOR/1
  "B "/1 -> XOR/2, AND/2
  XOR/1 -> Sum/1
  AND/1 -> Carry/1

== system UART/Rx Only/Baudrate Generator/BaudTimer1/Counter1/Half Adder5 ==
  A : Inport
  "B " : Inport  Port=2
  AND : Logic  IconShape=distinctive  AllPortsSameDT=off  OutDataTypeStr=boolean
  XOR : Logic  Operator=XOR  IconShape=distinctive  AllPortsSameDT=off  OutDataTypeStr=boolean
  Sum : Outport
  Carry : Outport  Port=2
  wires:
  A/1 -> AND/1, XOR/1
  "B "/1 -> XOR/2, AND/2
  XOR/1 -> Sum/1
  AND/1 -> Carry/1

== system UART/Rx Only/Baudrate Generator/BaudTimer1/Counter1/Half Adder6 ==
  A : Inport
  "B " : Inport  Port=2
  XOR : Logic  Operator=XOR  IconShape=distinctive  AllPortsSameDT=off  OutDataTypeStr=boolean
  Sum : Outport
  wires:
  A/1 -> XOR/1
  "B "/1 -> XOR/2
  XOR/1 -> Sum/1

== system UART/Rx Only/Baudrate Generator/BaudTimer1/Counter1/Half Adder7 ==
  A : Inport
  "B " : Inport  Port=2
  AND : Logic  IconShape=distinctive  AllPortsSameDT=off  OutDataTypeStr=boolean
  XOR : Logic  Operator=XOR  IconShape=distinctive  AllPortsSameDT=off  OutDataTypeStr=boolean
  Sum : Outport
  Carry : Outport  Port=2
  wires:
  A/1 -> AND/1, XOR/1
  "B "/1 -> XOR/2, AND/2
  XOR/1 -> Sum/1
  AND/1 -> Carry/1

== system UART/Rx Only/Baudrate Generator/BaudTimer1/TController/Prescaler_Controller1 ==
  StoreTReg : Inport
  TC : Inport  Port=2
  TReg : Inport  Port=3
  Enable : Inport  Port=4
  CLK : Inport  Port=5
  "CLR " : Inport  Port=6
  AND{,1..3} (4 alike) : Logic  IconShape=distinctive  AllPortsSameDT=off  OutDataTypeStr=boolean
  Delay One Step : Delay  DelayLength=1
  Demux : Demux  Outputs=8
  NOR : Logic  Operator=NOR  Inputs=8  IconShape=distinctive  AllPortsSameDT=off  OutDataTypeStr=boolean
  NOT : Logic  Operator=NOT  IconShape=distinctive  AllPortsSameDT=off  OutDataTypeStr=boolean
  NOT1 : Logic  Operator=NOT  IconShape=distinctive  AllPortsSameDT=off  OutDataTypeStr=boolean
  OR : Logic  Operator=OR  Inputs=3  IconShape=distinctive  AllPortsSameDT=off  OutDataTypeStr=boolean
  S-R Flip-Flop : simulink_extras/Flip Flops/S-R Flip-Flop  initial_condition=0
  Scope : Scope
      settings: ActiveDisplayYMinimum=-1  ActiveDisplayYMaximum=1  DataLoggingVariableName=ScopeData2
  XOR : Logic  Operator=XOR  IconShape=distinctive  AllPortsSameDT=off  OutDataTypeStr=boolean
  CLK_Next : Outport
  INC : Outport  Port=2
  TC_RST : Outport  Port=3
  wires:
  TReg/1 -> XOR/1
  Demux/1 -> NOR/1
  TC/1 -> XOR/2
  XOR/1 -> Demux/1
  Demux/2 -> NOR/2
  Demux/3 -> NOR/3
  Demux/4 -> NOR/4
  Demux/5 -> NOR/5
  Demux/6 -> NOR/6
  Demux/7 -> NOR/7
  Demux/8 -> NOR/8
  "CLR "/1 -> OR/3
  NOR/1 -> NOT/1, AND1/1
  Enable/1 -> AND1/2, AND/1
  OR/1 -> Delay One Step/1
  StoreTReg/1 -> OR/1
  AND/1 -> INC/1
  Delay One Step/1 -> AND3/1, TC_RST/1
  AND1/1 -> S-R Flip-Flop/1
  S-R Flip-Flop/1 -> AND2/2
  NOT/1 -> AND2/1
  AND2/1 -> OR/2, Scope/1, CLK_Next/1
  CLK/1 -> NOT1/1, AND/2
  AND3/1 -> S-R Flip-Flop/2
  NOT1/1 -> AND3/2

== matlab function UART/Subsystem/PC Tx/MATLAB Function ==
  data: u input; y output
function y = fcn(u)

y = 1/u;

== stateflow chart UART/Subsystem/PC Tx/Chart ==
  state Idle
    entry:
    CurrentBit=0;
    end
    during:
    Tx=Enable;
    end
  state Send_StartBit
    entry:
    Tx=0;
    end
  state Wait
  state Buffer
  state Send_Stop_bit
    entry:
    Tx=1
    end
  state Increase_Count
    entry:
    CurrentBit = CurrentBit + 1;
    % Access the CurrentBit-th bit of Bits
    Tx = Bits(9-CurrentBit);  % For vector Bits
    end
  (default) -> Idle
  Send_Stop_bit -> Idle : after(Baudrate,sec)
  Idle -> Send_StartBit : [Send==1]
  Send_StartBit -> Wait
  Increase_Count -> Wait : [CurrentBit <=8]
  Wait -> Buffer : after(Baudrate,sec)
  Buffer -> Send_Stop_bit [order 1] : [CurrentBit>=8]
  Buffer -> Increase_Count [order 2] : [CurrentBit<8]
  data: Baudrate input; Send input; Bits input; Enable input; Tx output; CurrentBit local

== stateflow chart UART/Subsystem/PC RX/Chart ==
  state WaitStartBitle
    entry:
    CurrentBit=0;
    end
  state ClearBuffer
    entry:
    Buffer = zeros(8, 1);
  state Wait
  state Buffer
  state ReceieveStopBit
  state Increase_Count
    entry:
    CurrentBit = CurrentBit + 1;
    if CurrentBit <= 8
    % Store the current value of Rx in the Buffer at CurrentBit-th position
    Buffer(9-CurrentBit) = Rx;
    else
    % Handle out-of-bounds case (optional)
    error('CurrentBit exceeds the valid range.');
    end
    end
  (default) -> WaitStartBitle
  ReceieveStopBit -> WaitStartBitle : after(Baudrate,sec)
  WaitStartBitle -> ClearBuffer : [Rx==0&&Enable==1]
  ClearBuffer -> Wait
  Increase_Count -> Wait : [CurrentBit <=8]
  Wait -> Buffer : after(Baudrate,sec)
  Buffer -> ReceieveStopBit [order 1] : [CurrentBit>=8]
  Buffer -> Increase_Count [order 2] : [CurrentBit<8]
  data: Baudrate input; Enable input; Buffer output; CurrentBit local; Rx input

== matlab function UART/Subsystem/PC RX/MATLAB Function ==
  data: u input; y output
function y = fcn(u)

y = 1/u;

== stateflow chart UART/Chart ==
  state LoadBR
    entry:
    Data = 1;
    CLR = 0;
    StoreBR = 1;
  state Startup
    entry:
    Data = 0;
    CLR = 1;
  state Wait
    entry:
    StoreBR = 0;
  state End
    entry:
    StorePS = 0;
    EN_UART = 1;
  state LoadPS
    entry:
    StorePS = 1;
    Data = 0;
  state END
    entry:
    Data = 0;
  (default) -> Startup
  LoadBR -> Wait : [CLK==1]
  Startup -> LoadBR : [CLK==0]
  Wait -> LoadPS : [CLK == 0]
  LoadPS -> End : [CLK ==1]
  End -> END : [CLK==0]
  data: CLR output; Data output; StoreBR output; StorePS output; CLK input; EN_UART output

== stateflow chart UART/Chart1 ==
  state Startup
    Data = 0;
    StoreTx=0;
    Send=0;
  state StartSend
  state LoadTx
    entry:
    Data = ToSend;
    StoreTx = 1;
  state END1
    entry:
    Send=1;
  state Wait
    entry:
    StoreTx=0;
    Data = 0;
  (default) -> Startup
  END1 -> Startup : [CLK==1&&StartSend==0]
  Startup -> StartSend : [StartSend == 1]
  StartSend -> LoadTx : [CLK==0]
  LoadTx -> Wait : [CLK==1]
  Wait -> END1 : [CLK==0]
  data: Data output; CLK input; ToSend input; StoreTx output; Send output; StartSend input

== matlab function UART/MATLAB Function ==
  data: baudrate input; transmission output; byte_data input; transmit input
function transmission = uart_transmitter(baudrate, byte_data, transmit)
% UART Transmitter Function
% Inputs:
%   baudrate - transmission speed (bits per second)
%   byte_data - 8-bit data to transmit (0-255)
%   transmit - trigger bit (1 to start transmission, 0 for idle)
% Output:
%   transmission - current bit being transmitted (scalar double)

% Persistent variables to maintain state between function calls
persistent bit_counter;
persistent frame_data;
persistent bit_timer;
persistent transmitting;
persistent sample_time;

% Initialize persistent variables on first call
if isempty(bit_counter)
    bit_counter = uint8(0);
    frame_data = zeros(1,10); % Pre-allocate for 10 bits (start + 8 data + stop)
    bit_timer = uint32(0);
    transmitting = false;
    sample_time = 5e-6; % 5 microseconds - adjust to match your Simulink model sample time
end

% Calculate bit period from baudrate
bit_period = 1.0 / double(baudrate);
samples_per_bit = uint32(bit_period / sample_time);

% Default output (idle high) - ensure it's a scalar double
transmission = double(1);

% Start transmission when transmit goes high
if transmit && ~transmitting
    % Create UART frame: [start_bit, data_bits(LSB first), stop_bit]
    
    % Convert byte to bits (LSB first)
    temp_byte = uint8(byte_data);
    
    % Start bit (0)
    frame_data(1) = 0;
    
    % Data bits (LSB first)
    for i = 1:8
        frame_data(i+1) = double(mod(temp_byte, 2));
        temp_byte = bitshift(temp_byte, -1);
    end
    
    % Stop bit (1)
    frame_data(10) = 1;
    
    % Reset counters and start transmitting
    bit_counter = uint8(1);
    bit_timer = uint32(0);
    transmitting = true;
end

% Handle ongoing transmission
if transmitting
    % Output current bit
    if bit_counter <= 10
        transmission = double(frame_data(bit_counter));
    else
        transmission = double(1); % Idle high after transmission
    end
    
    % Update bit timer
    bit_timer = bit_timer + uint32(1);
    
    % Check if it's time for next bit
    if bit_timer >= samples_per_bit
        bit_timer = uint32(0);
        bit_counter = bit_counter + uint8(1);
        
        % Check if transmission is complete
        if bit_counter > uint8(10)
            transmitting = false;
            bit_counter = uint8(0);
        end
    end
end

end
